simulink model "AM2"  (R2021a)
settings: Solver=VariableStepAuto  StartTime=0.0  StopTime=20  RelTol=1e-3
libraries: commanapbnd3 x1
settings Model: Creator=Devraj Kashyap  LastModifiedBy=Devraj Kashyap

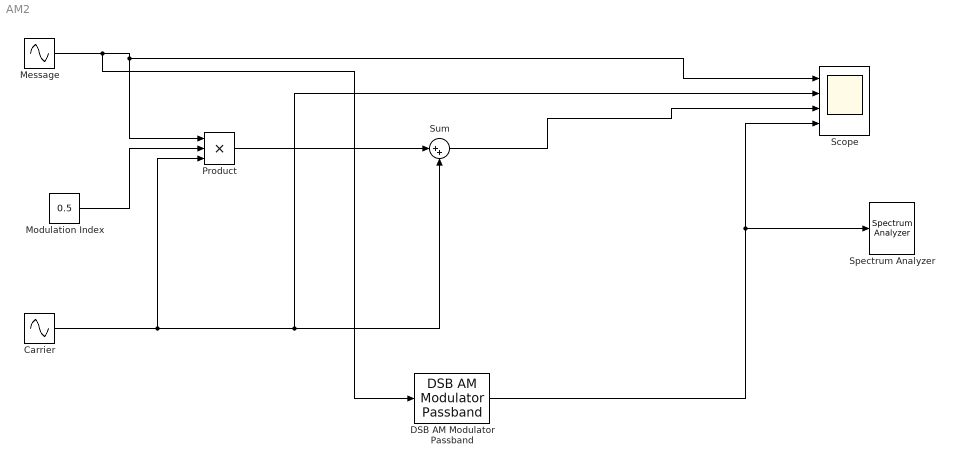
== system AM2 ==
  Carrier : Sin  Frequency=2*pi*50  Phase=90  SampleTime=0.001
  DSB AM Modulator Passband : commanapbnd3/DSB AM Modulator Passband  Fc=100  Ph=0  Offset=1
      settings: SourceProductBaseCode=CM
  Message : Sin  Frequency=2*pi*5  Samples=100  SampleTime=0.001
  Modulation Index : Constant  Value=0.5
  Product : Product  Inputs=3
  Scope : Scope  NumInputPorts=4
  Spectrum Analyzer : SpectrumAnalyzer
  Sum : Sum  Inputs=|++
  wires:
  Message/1 -> DSB AM Modulator Passband/1, Product/1, Scope/1
  Modulation Index/1 -> Product/2
  Product/1 -> Sum/1
  Carrier/1 -> Product/3, Sum/2, Scope/2
  Sum/1 -> Scope/3
  DSB AM Modulator Passband/1 -> Spectrum Analyzer/1, Scope/4
